simulink model "ComplexPhaseDetectorDual"  (R2016a)
settings: Solver=VariableStepAuto  StartTime=0.0  StopTime=.05  RelTol=1e-6
PreLoadFcn:
  | Bits = 4
  | Ts=2*3/280e6
  | dBRange=11
  | maxNumErrs=500
  | maxNumBits=1e6
  | AM_Gain=AM_GainDiff;
  | AGC_Gain=AGC_GainCalc;
  | load('IIR_Coeffs.mat');
InitFcn:
  | Br= 1/(10*Ts)
  | FreqOffset=00
  | Mode=2
  | BitsPer=[2,2,1,1]
  | EbNo=50
  | N=6
undefined symbols (not defined in the file or in its folder): designMultirateFIR, DiscIntNeverNeededParam
libraries: xbsIndex_r4 x1085, commfilt2 x12, commsink2 x6, dspsigops x5, dspmlti4 x2, commrfcorlib x2, commchan3 x2, dspfdesign x2, dspstat3 x2, commdigbbndpm3 x1, commrandsrc3 x1
(part 2 of 13)

== system ComplexPhaseDetectorDual/AD9957 ==
  In1 : Inport
  Add3 : Sum
  Complex to Real-Imag3 : ComplexToRealImag
  FIR Interpolation : dspmlti4/FIR Interpolation  FilterSource=Auto  h=designMultirateFIR(3,1)  L=8  FilterObject=FINTERP  framing=Allow multirate processing  outputBufInitCond=0  roundingMode=Floor  overflowMode=off  firstCoeffDataTypeStr=Inherit: Same word length as input  firstCoeffMin=[]  firstCoeffMax=[]  firstCoeffLastDataTypeStr=Inherit: Same word length as input  outputDataTypeStr=Inherit: Same as accumulator  outputMin=[]  outputMax=[]  outputLastDataTypeStr=Inherit: Same as accumulator
  NCO : dspsigops/NCO  AccIncSrc=Specify via dialog  AccInc=16384*3/8  PhaseOffsetSrc=Specify via dialog  PhaseOffset=0  AccumWL=16  HasDither=off  DitherWL=4  PNgeneratorLength=19  HasPhaseQuantizer=off  TableDepth=12  HasOutputPhaseError=off  Formula=Sine and cosine  DataType=double  OutputWL=16  OutputFL=14  CompMethod=Table lookup (no interpolation)  SampleTime=Ts/8  SamplesPerFrame=1  OutputFrames=off
  PhaseDetect1 : Product
  PhaseDetect2 : Product
  Out1 : Outport
  wires:
  In1/1 -> FIR Interpolation/1
  NCO/1 -> PhaseDetect2/2
  Complex to Real-Imag3/1 -> PhaseDetect1/1
  PhaseDetect2/1 -> Add3/1
  PhaseDetect1/1 -> Add3/2
  Complex to Real-Imag3/2 -> PhaseDetect2/1
  FIR Interpolation/1 -> Complex to Real-Imag3/1
  NCO/2 -> PhaseDetect1/2
  Add3/1 -> Out1/1

== system ComplexPhaseDetectorDual/AD9957-2 ==
  In1 : Inport
  Add3 : Sum
  Complex to Real-Imag3 : ComplexToRealImag
  FIR Interpolation : dspmlti4/FIR Interpolation  FilterSource=Auto  h=designMultirateFIR(3,1)  L=8  FilterObject=FINTERP  framing=Allow multirate processing  outputBufInitCond=0  roundingMode=Floor  overflowMode=off  firstCoeffDataTypeStr=Inherit: Same word length as input  firstCoeffMin=[]  firstCoeffMax=[]  firstCoeffLastDataTypeStr=Inherit: Same word length as input  outputDataTypeStr=Inherit: Same as accumulator  outputMin=[]  outputMax=[]  outputLastDataTypeStr=Inherit: Same as accumulator
  NCO : dspsigops/NCO  AccIncSrc=Specify via dialog  AccInc=16384*3/8  PhaseOffsetSrc=Specify via dialog  PhaseOffset=0  AccumWL=16  HasDither=off  DitherWL=4  PNgeneratorLength=19  HasPhaseQuantizer=off  TableDepth=12  HasOutputPhaseError=off  Formula=Sine and cosine  DataType=double  OutputWL=16  OutputFL=14  CompMethod=Table lookup (no interpolation)  SampleTime=Ts/8  SamplesPerFrame=1  OutputFrames=off
  PhaseDetect1 : Product
  PhaseDetect2 : Product
  Out1 : Outport
  wires:
  Add3/1 -> Out1/1
  NCO/2 -> PhaseDetect1/2
  FIR Interpolation/1 -> Complex to Real-Imag3/1
  Complex to Real-Imag3/2 -> PhaseDetect2/1
  PhaseDetect1/1 -> Add3/2
  PhaseDetect2/1 -> Add3/1
  Complex to Real-Imag3/1 -> PhaseDetect1/1
  NCO/1 -> PhaseDetect2/2
  In1/1 -> FIR Interpolation/1

== system ComplexPhaseDetectorDual/AGCtoAWGN1 ==
  AGC : Inport
  Bias2 : Bias  Bias=100
  Gain10 : Gain  Gain=3.55
  Gain9 : Gain  Gain=-1/10
  Math Function : Math  Operator=10^u  SaturateOnIntegerOverflow=on
  Variance : Outport
  wires:
  Math Function/1 -> Gain10/1
  Gain10/1 -> Variance/1
  Gain9/1 -> Math Function/1
  Bias2/1 -> Gain9/1
  AGC/1 -> Bias2/1

== system ComplexPhaseDetectorDual/AGCtoAWGN2 ==
  AGC : Inport
  Bias2 : Bias  Bias=100
  Gain10 : Gain  Gain=3.55
  Gain9 : Gain  Gain=-1/10
  Math Function : Math  Operator=10^u  SaturateOnIntegerOverflow=on
  Variance : Outport
  wires:
  AGC/1 -> Bias2/1
  Bias2/1 -> Gain9/1
  Gain9/1 -> Math Function/1
  Gain10/1 -> Variance/1
  Math Function/1 -> Gain10/1

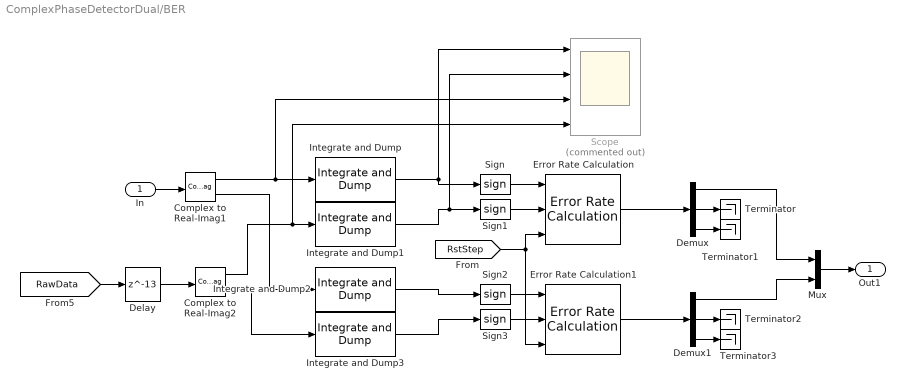
== system ComplexPhaseDetectorDual/BER ==
  In : Inport
  Complex to Real-Imag1 : ComplexToRealImag
  Complex to Real-Imag2 : ComplexToRealImag
  Delay : Delay  DelayLength=13
  Demux : Demux  Outputs=3
  Demux1 : Demux  Outputs=3
  Error Rate Calculation : commsink2/Error Rate Calculation  N=0  st_delay=100  cp_mode=Entire frame  subframe=[]  PMode=Port  WsName=BER  RsMode2=on  stop=off  numErr=maxNumErrs  maxBits=maxNumBits
  Error Rate Calculation1 : commsink2/Error Rate Calculation  N=0  st_delay=100  cp_mode=Entire frame  subframe=[]  PMode=Port  WsName=BER  RsMode2=on  stop=off  numErr=maxNumErrs  maxBits=maxNumBits
  Integrate and Dump{,1..3} (4 alike) : commfilt2/Integrate and Dump  obssamples=1/(Br*Ts)  offsetsamples=3  nodump=off  roundingMode=Floor  overflowMode=off  outputDataTypeStr=Inherit: Same as accumulator  outputLastDataTypeStr=Inherit: Same as accumulator
  Mux : Mux  Inputs=2
  Scope : Scope  Commented=on  NumInputPorts=4
  Sign{,1..3} (4 alike) : Signum
  Terminator{,1..3} (4 alike) : Terminator
  Out1 : Outport
  wires:
  Integrate and Dump1/1 -> Scope/2, Sign1/1
  Error Rate Calculation/1 -> Demux/1
  Integrate and Dump/1 -> Scope/1, Sign/1
  Sign/1 -> Error Rate Calculation/1
  Sign1/1 -> Error Rate Calculation/2
  In/1 -> Complex to Real-Imag1/1
  Complex to Real-Imag2/1 -> Scope/4, Integrate and Dump1/1
  Delay/1 -> Complex to Real-Imag2/1
  [RawData] -> Delay/1
  Complex to Real-Imag1/1 -> Scope/3, Integrate and Dump/1
  Integrate and Dump3/1 -> Sign3/1
  Error Rate Calculation1/1 -> Demux1/1
  Integrate and Dump2/1 -> Sign2/1
  Sign2/1 -> Error Rate Calculation1/1
  Sign3/1 -> Error Rate Calculation1/2
  Complex to Real-Imag2/2 -> Integrate and Dump3/1
  [RstStep] -> Error Rate Calculation1/3, Error Rate Calculation/3
  Complex to Real-Imag1/2 -> Integrate and Dump2/1
  Demux/1 -> Mux/1
  Demux1/1 -> Mux/2
  Demux/2 -> Terminator/1
  Demux/3 -> Terminator1/1
  Demux1/2 -> Terminator2/1
  Demux1/3 -> Terminator3/1
  Mux/1 -> Out1/1

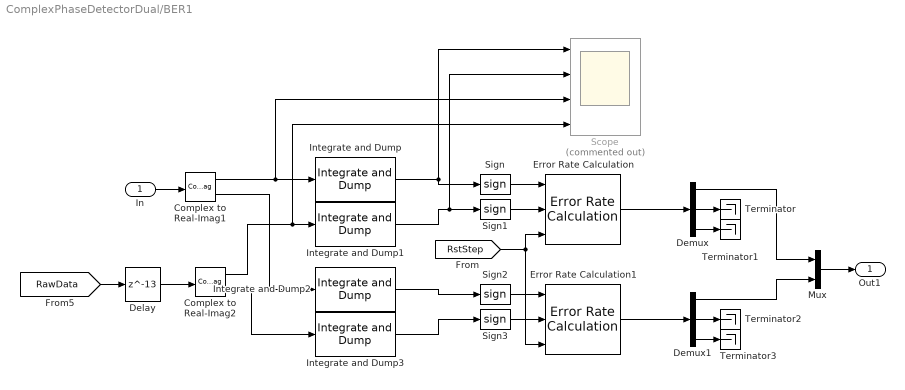
== system ComplexPhaseDetectorDual/BER1 ==
  In : Inport
  Complex to Real-Imag1 : ComplexToRealImag
  Complex to Real-Imag2 : ComplexToRealImag
  Delay : Delay  DelayLength=13
  Demux : Demux  Outputs=3
  Demux1 : Demux  Outputs=3
  Error Rate Calculation : commsink2/Error Rate Calculation  N=0  st_delay=100  cp_mode=Entire frame  subframe=[]  PMode=Port  WsName=BER  RsMode2=on  stop=off  numErr=maxNumErrs  maxBits=maxNumBits
  Error Rate Calculation1 : commsink2/Error Rate Calculation  N=0  st_delay=100  cp_mode=Entire frame  subframe=[]  PMode=Port  WsName=BER  RsMode2=on  stop=off  numErr=maxNumErrs  maxBits=maxNumBits
  Integrate and Dump{,1..3} (4 alike) : commfilt2/Integrate and Dump  obssamples=1/(Br*Ts)  offsetsamples=3  nodump=off  roundingMode=Floor  overflowMode=off  outputDataTypeStr=Inherit: Same as accumulator  outputLastDataTypeStr=Inherit: Same as accumulator
  Mux : Mux  Inputs=2
  Scope : Scope  Commented=on  NumInputPorts=4
  Sign{,1..3} (4 alike) : Signum
  Terminator{,1..3} (4 alike) : Terminator
  Out1 : Outport
  wires:
  Mux/1 -> Out1/1
  Demux1/3 -> Terminator3/1
  Demux1/2 -> Terminator2/1
  Demux/3 -> Terminator1/1
  Demux/2 -> Terminator/1
  Demux1/1 -> Mux/2
  Demux/1 -> Mux/1
  Complex to Real-Imag1/2 -> Integrate and Dump2/1
  [RstStep] -> Error Rate Calculation/3, Error Rate Calculation1/3
  Complex to Real-Imag2/2 -> Integrate and Dump3/1
  Sign3/1 -> Error Rate Calculation1/2
  Sign2/1 -> Error Rate Calculation1/1
  Integrate and Dump2/1 -> Sign2/1
  Error Rate Calculation1/1 -> Demux1/1
  Integrate and Dump3/1 -> Sign3/1
  Complex to Real-Imag1/1 -> Integrate and Dump/1, Scope/3
  [RawData] -> Delay/1
  Delay/1 -> Complex to Real-Imag2/1
  Complex to Real-Imag2/1 -> Integrate and Dump1/1, Scope/4
  In/1 -> Complex to Real-Imag1/1
  Sign1/1 -> Error Rate Calculation/2
  Sign/1 -> Error Rate Calculation/1
  Integrate and Dump/1 -> Sign/1, Scope/1
  Error Rate Calculation/1 -> Demux/1
  Integrate and Dump1/1 -> Sign1/1, Scope/2

== system ComplexPhaseDetectorDual/Conjugate ==
  In1 : Inport
  Complex to Real-Imag : ComplexToRealImag
  Real-Imag to Complex : RealImagToComplex
  Unary Minus : UnaryMinus
  Out1 : Outport
  wires:
  In1/1 -> Complex to Real-Imag/1
  Complex to Real-Imag/1 -> Real-Imag to Complex/1
  Complex to Real-Imag/2 -> Unary Minus/1
  Unary Minus/1 -> Real-Imag to Complex/2
  Real-Imag to Complex/1 -> Out1/1

== system ComplexPhaseDetectorDual/Knob ==

== system ComplexPhaseDetectorDual/LockImag ==
  In : Inport
  Sub : Inport  Port=2
  Rst_n : Inport  Port=3
  Constant : xbsIndex_r4/Constant  const=0  gui_display_data_type=Fixed-point  arith_type=Unsigned  n_bits=13  bin_pt=0  preci_type=Single  exp_width=8  frac_width=24  explicit_period=off  period=1  equ=P=C  opselect=C  inp2=PCIN>>17  opr=+  inp1=P  carry=CIN  dbl_ovrd=off  block_type=constant
  LockReal : xbsIndex_r4/AddSub  mode=Addition or Subtraction  use_carryin=off  use_carryout=off  en=off  latency=1  precision=User Defined  arith_type=Unsigned  n_bits=13  bin_pt=0  quantization=Truncate  overflow=Saturate  use_behavioral_HDL=off  hw_selection=Fabric  pipelined=off  dbl_ovrd=off  block_type=addsub
  Mux : xbsIndex_r4/Mux  inputs=2  en=off  latency=0  precision=Full  arith_type=Unsigned  n_bits=16  bin_pt=14  quantization=Truncate  overflow=Wrap  dbl_ovrd=off  block_type=mux
  Out : Outport
  wires:
  Rst_n/1 -> Mux/1
  Constant/1 -> Mux/2
  Mux/1 -> LockReal/1
  LockReal/1 -> Out/1, Mux/3
  Sub/1 -> LockReal/3
  In/1 -> LockReal/2

== system ComplexPhaseDetectorDual/LockReal ==
  In : Inport
  Sub : Inport  Port=2
  Rst_n : Inport  Port=3
  Constant : xbsIndex_r4/Constant  const=0  gui_display_data_type=Fixed-point  arith_type=Unsigned  n_bits=13  bin_pt=0  preci_type=Single  exp_width=8  frac_width=24  explicit_period=off  period=1  equ=P=C  opselect=C  inp2=PCIN>>17  opr=+  inp1=P  carry=CIN  dbl_ovrd=off  block_type=constant
  LockReal : xbsIndex_r4/AddSub  mode=Addition or Subtraction  use_carryin=off  use_carryout=off  en=off  latency=1  precision=User Defined  arith_type=Unsigned  n_bits=13  bin_pt=0  quantization=Truncate  overflow=Saturate  use_behavioral_HDL=off  hw_selection=Fabric  pipelined=off  dbl_ovrd=off  block_type=addsub
  Mux : xbsIndex_r4/Mux  inputs=2  en=off  latency=0  precision=Full  arith_type=Unsigned  n_bits=16  bin_pt=14  quantization=Truncate  overflow=Wrap  dbl_ovrd=off  block_type=mux
  Out : Outport
  wires:
  In/1 -> LockReal/2
  Sub/1 -> LockReal/3
  LockReal/1 -> Mux/3, Out/1
  Mux/1 -> LockReal/1
  Constant/1 -> Mux/2
  Rst_n/1 -> Mux/1

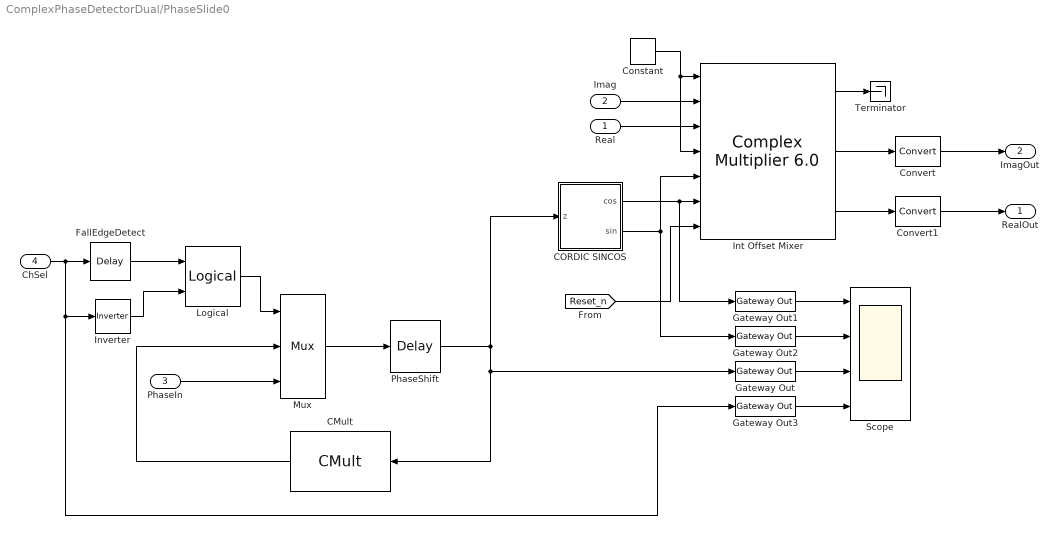
== system ComplexPhaseDetectorDual/PhaseSlide0 ==
  Real : Inport
  Imag : Inport  Port=2
  PhaseIn : Inport  Port=3
  ChSel : Inport  Port=4
  CMult : xbsIndex_r4/CMult  const=.999  gui_display_data_type=Fixed-point  const_n_bits=18  const_bin_pt=17  float_type=Single  exp_bits=8  fraction_bits=24  en=off  latency=1  precision=User Defined  arith_type="Signed  (2's comp)"  n_bits=21  bin_pt=17  quantization=Truncate  overflow=Wrap  use_behavioral_HDL=off  mem_type=Distributed RAM  pipeline=off  dbl_ovrd=off  block_type=cmult
  CORDIC SINCOS : Subsystem  mask(Xilinx CORDIC SINCOS){stages=17, pe_nbits=21, pe_binpt=17, pipeline_x=ones(1,17), prev_stages=17, pipeline=[1  1  1  1  1  1  1  1  1  1  1  1  1  1  1  1  1]}
      mask prompts: stages "Number of Processing Elements (integer value starting from 1)"; pe_nbits "Input Data Width"; pe_binpt "Input Binary Point Position"; pipeline_x "Latency for each Processing Element [1 0 0 1]"; prev_stages "Previous Number of Stages"; pipeline "Previous Pipeline Values"
      mask help: A parallel implementation, circular rotation mode CORDIC processor for calculating Sine and Cosine of input angle z. The number of iteration stages (and resultant output accuracy) and the processor arithmetic precision are controlled by the mask customization.
      mask init:
      | [bg,fg] = xlcmap('XBlock',0);
      | iPos = get_param(gcb,'Position');
      | iWidth=iPos(3)-iPos(1); iHeight=iPos(4)-iPos(2);
      | iCx=iWidth/2;
      | iCy=iHeight/2;
      | [logoX, logoY] = xlogo(iPos);
      | sav_gcb=gcb;
      | stages = round(sum(abs(stages)));
      | if (stages == 0)
      | 	stages = prev_stages;
      | end
      | x = zeros(1,stages);
      | pipe_size = max(size(pipeline_x));
      | if pipe_size >= stages
      | 	x(1,1:stages) = pipeline_x(1,1:stages);
      | else
      | 	x(1,1:pipe_size) = pipeline_x(1,1:pipe_size);
      | end
      | 
      | if (stages ~=prev_stages)
      | 	pipeline=x;
      | 	cordic_pe = find_system(gcb, 'lookUnderMasks', 'all', 'FollowLinks','on','masktype', 'CORDIC parallel PE');
      |     
      |   a=find_system(cordic_pe{1}, 'lookUnderMasks', 'all', 'FollowLinks','on','masktype', 'CORDIC iteration PE');
      |   for i= 2:length(a)
      |     for j=1:3
      | 	  delete_line(cordic_pe{1}, ['CORDIC PE' int2str(i-1) '/' int2str(j)], ['CORDIC PE' int2str(i) '/' int2str(j)]);
      |     end
      |   end
      |     if length(a)>0,
      |       delete_line(cordic_pe{1}, 'x/1', 'CORDIC PE1/1');
      |       delete_line(cordic_pe{1}, 'y/1', 'CORDIC PE1/2');
      |       delete_line(cordic_pe{1}, 'z/1', 'CORDIC PE1/3');
      |       delete_line(cordic_pe{1}, ['CORDIC PE' int2str(length(a)) '/1'],'X/1');
      |       delete_line(cordic_pe{1}, ['CORDIC PE' int2str(length(a)) '/2'],'Y/1');
      |       delete_line(cordic_pe{1}, ['CORDIC PE' int2str(length(a)) '/3'],'Terminator/1');
      |     elseif length(a)==0
      |       temp_port=get_param([cordic_pe{1} '/x'],'porthandles');
      |       temp_line=get_param(temp_port.Outport,'line');
      |       if temp_line>=0  delete_line(temp_line); end
      |       temp_port=get_param([cordic_pe{1} '/y'],'porthandles');
      |       temp_line=get_param(temp_port.Outport,'line');
      |       if temp_line>=0  delete_line(temp_line); end
      |       temp_port=get_param([cordic_pe{1} '/z'],'porthandles');
      |       temp_line=get_param(temp_port.Outport,'line');
      |       if temp_line>=0  delete_line(temp_line); end
      |     end
      | 
      |     for i=2:length(a)
      |       delete_block(a{i});
      |     end
      |     for i=2:stages,
      |         add_block([cordic_pe{1} '/CORDIC PE1'], [cordic_pe{1} '/CORDIC PE' int2str(i)], 'ii', int2str(i-1),'pe_nbits', 'pe_nbits','pe_binpt', 'pe_binpt','pipeline',['pipeline(1,' int2str(i) ')'],'position',[150+(i-1)*125, 70, 205+(i-1)*125, 130]);
      |     end
      | 
      |     for i= 2:stages,
      |       for j=1:3
      | 		add_line(cordic_pe{1}, ['CORDIC PE' int2str(i-1) '/' int2str(j)], ['CORDIC PE' int2str(i) '/' int2str(j)], 'autorouting', 'on');
      |       end
      |     end
      | 
      |     if stages==0
      |       add_line(cordic_pe{1}, 'x/1', 'X/1', 'autorouting', 'on');
      |       add_line(cordic_pe{1}, 'y/1', 'Terminator/1', 'autorouting', 'on');
      |       add_line(cordic_pe{1}, 'z/1', 'Z/1', 'autorouting', 'on');
      |     elseif stages>0
      |       add_line(cordic_pe{1}, 'x/1', 'CORDIC PE1/1', 'autorouting', 'on');
      |       add_line(cordic_pe{1}, 'y/1', 'CORDIC PE1/2', 'autorouting', 'on');
      |       add_line(cordic_pe{1}, 'z/1', 'CORDIC PE1/3', 'autorouting', 'on');
      | 
      |       set_param([cordic_pe{1} '/' 'X'], 'Position', [150+stages*125, 72, 180+stages*125, 86]);
      |       set_param([cordic_pe{1} '/' 'Y'], 'Position', [210+stages*125, 92, 225+stages*125, 108]);
      |       set_param([cordic_pe{1} '/' 'Terminator'], 'Position', [240+stages*125, 113, 270+stages*125, 127]);
      | 
      |       add_line(cordic_pe{1}, ['CORDIC PE' int2str(stages) '/1'], 'X/1', 'autorouting', 'on');
      |       add_line(cordic_pe{1}, ['CORDIC PE' int2str(stages) '/2'], 'Y/1', 'autorouting', 'on');
      |       add_line(cordic_pe{1}, ['CORDIC PE' int2str(stages) '/3'],'Terminator/1', 'autorouting', 'on');
      | 
      |       % force a "compile" of the constituent constant blocks to
      |       % workaround a data propagation problem
      |       find_system(cordic_pe{1}, 'lookUnderMasks', 'all', 'FollowLinks', 'on', 'MaskType','Xilinx Constant Block');
      |   end
      | 	set_param(sav_gcb, 'prev_stages', int2str(stages));
      | 	set_param(sav_gcb, 'pipeline', [ '[' int2str(x) ']']);
      | else
      | 	if (sum(pipeline~=x))
      | 		set_param(gcb, 'pipeline', [ '[' int2str(x) ']']);
      | 	end
      | end
      | str = sprintf('-%d',sum(x) + 3);
      settings: CopyFcn=set_param(gcb, 'MaskSelfModifiable', 'on', 'LinkStatus', 'none');
      mask Help: eval('');xlDoc('-book','sysgen','-topic','CORDIC_SINCOS');
      mask Display:
      | patch([0 iWidth iWidth 0],[0 0 iHeight iHeight] , bg);
      | patch(logoX,logoY , fg);
      | text(iCx-6,iCy,'z');
      | text(iCx,iCy+4,str);
      | port_label('input',1,'z');
      | port_label('output',1,'cos');
      | port_label('output',2,'sin');
      | plot([0 0 iWidth iWidth 0], [0 iHeight iHeight 0 0]);
  Constant : xbsIndex_r4/Constant  const=1  gui_display_data_type=Boolean  arith_type=Boolean  n_bits=16  bin_pt=14  preci_type=Single  exp_width=8  frac_width=24  explicit_period=on  period=Ts  equ=P=C  opselect=C  inp2=PCIN>>17  opr=+  inp1=P  carry=CIN  dbl_ovrd=off  block_type=constant
  Convert : xbsIndex_r4/Convert  gui_display_data_type=Fixed-point  arith_type="Signed  (2's comp)"  n_bits=18  bin_pt=17  float_type=Single  exp_bits=8  fraction_bits=24  quantization=Truncate  overflow=Saturate  en=off  latency=1  pipeline=off  dbl_ovrd=off  block_type=convert
  Convert1 : xbsIndex_r4/Convert  gui_display_data_type=Fixed-point  arith_type="Signed  (2's comp)"  n_bits=18  bin_pt=17  float_type=Single  exp_bits=8  fraction_bits=24  quantization=Truncate  overflow=Saturate  en=off  latency=1  pipeline=off  dbl_ovrd=off  block_type=convert
  FallEdgeDetect : xbsIndex_r4/Delay  rst=off  infoeditControl=Selection of Reset will increase slice count due to use of real FFs and instead of SRLs  en=off  latency=4  reg_retiming=off  dbl_ovrd=off  block_type=delay
  Gateway Out{,1..3} (4 alike) : xbsIndex_r4/Gateway Out  inherit_from_input=off  hdl_port=off  rows=1  columns=1  UseAsDAC=off  DACChannel='1'  interface=None  automatic_assignment=on  address_offset=hex2dec('00')  intf_name=''  intf_description=''  timing_constraint=None  locs_specified=off  LOCs={}  io_standard={}  block_type=gatewayout
  Int Offset Mixer : xbsIndex_r4/Complex Multiplier 6.0   hasatlast=off  hasatuser=off  atuserwidth=1  hasbtlast=off  hasbtuser=off  btuserwidth=1  multtype=Use_Mults  optimizegoal=Resources  flowcontrol=NonBlocking  outputwidth=20  roundmode=Truncate  hasctrltlast=off  hasctrltuser=off  ctrltuserwidth=1  outtlastbehv=Null  latencyconfig=Manual  minimumlatency=3  aclken=off  aresetn=on  trim_axipin_name=on  simulation_type=hybrid_sim  simulation_model=sysgen:cmpy_v6_0  data_path_portlist={ 's_axis_a_tdata_real', 's_axis_a_tdata_imag', 's_axis_b_tdata_real', 's_axis_b_tdata_imag', 's_axis_ctrl_tdata_rounding_bit', 'm_axis_dout_tdata_real', 'm_axis_dout_tdata_imag' }  aportwidth=63  bportwidth=63  ip_name=Complex Multiplier  ip_version=6.0  dsptool_ready=true  ipcore_usecache=true  ipcore_useipmodelcache=true  ipcore_verbose=false  ipcore_latency_parameter='minimumlatency'  wrapper_available=true  port_translation_map={ 'aclken' => 'en', 'aresetn' => 'rst'}  block_type=cmpy_v6_0
  Inverter : xbsIndex_r4/Inverter  en=off  latency=0  dbl_ovrd=off  block_type=inv
  Logical : xbsIndex_r4/Logical  logical_function=AND  inputs=2  en=off  latency=0  precision=Full  arith_type=Unsigned  n_bits=16  bin_pt=0  align_bp=on  dbl_ovrd=off  block_type=logical
  Mux : xbsIndex_r4/Mux  inputs=2  en=off  latency=0  precision=Full  arith_type=Unsigned  n_bits=16  bin_pt=14  quantization=Truncate  overflow=Wrap  dbl_ovrd=off  block_type=mux
  PhaseShift : xbsIndex_r4/Delay  rst=off  infoeditControl=Selection of Reset will increase slice count due to use of real FFs and instead of SRLs  en=off  latency=1  reg_retiming=off  dbl_ovrd=off  block_type=delay
  Scope : Scope  NumInputPorts=4
  Terminator : Terminator
  RealOut : Outport
  ImagOut : Outport  Port=2
  wires:
  Imag/1 -> Int Offset Mixer/2
  Constant/1 -> Int Offset Mixer/4, Int Offset Mixer/1
  CORDIC SINCOS/2(sin) -> Int Offset Mixer/5, Gateway Out2/1
  Int Offset Mixer/1 -> Terminator/1
  Convert1/1 -> RealOut/1
  Real/1 -> Int Offset Mixer/3
  Convert/1 -> ImagOut/1
  CORDIC SINCOS/1(cos) -> Int Offset Mixer/6, Gateway Out1/1
  Mux/1 -> PhaseShift/1
  CMult/1 -> Mux/2
  PhaseIn/1 -> Mux/3
  ChSel/1 -> Gateway Out3/1, Inverter/1, FallEdgeDetect/1
  Logical/1 -> Mux/1
  FallEdgeDetect/1 -> Logical/1
  Inverter/1 -> Logical/2
  Gateway Out1/1 -> Scope/1
  Gateway Out2/1 -> Scope/2
  Gateway Out/1 -> Scope/3
  PhaseShift/1 -> CMult/1, Gateway Out/1, CORDIC SINCOS/1(z)
  Int Offset Mixer/3 -> Convert1/1
  Int Offset Mixer/2 -> Convert/1
  [Reset_n] -> Int Offset Mixer/7
  Gateway Out3/1 -> Scope/4

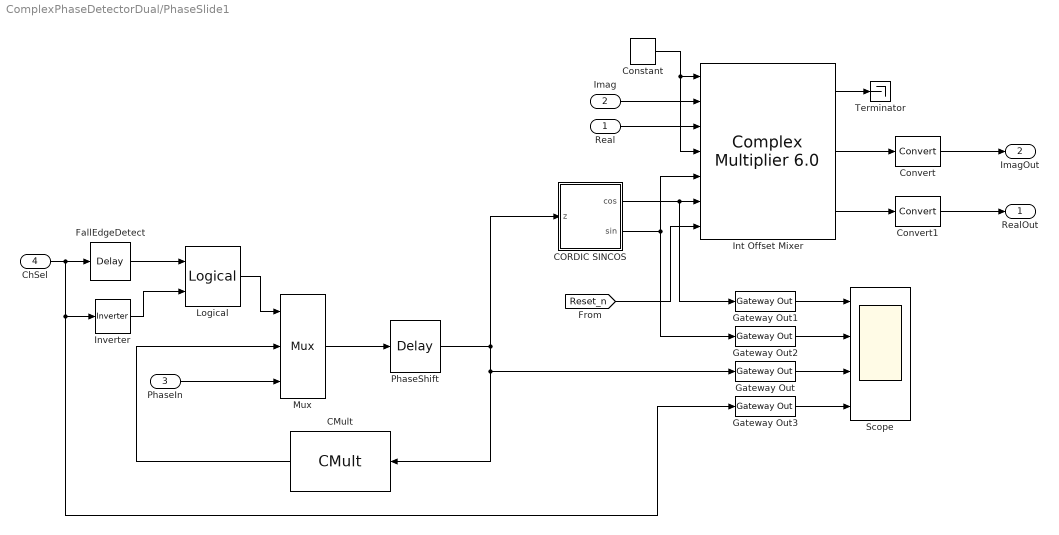
== system ComplexPhaseDetectorDual/PhaseSlide1 ==
  Real : Inport
  Imag : Inport  Port=2
  PhaseIn : Inport  Port=3
  ChSel : Inport  Port=4
  CMult : xbsIndex_r4/CMult  const=.999  gui_display_data_type=Fixed-point  const_n_bits=18  const_bin_pt=17  float_type=Single  exp_bits=8  fraction_bits=24  en=off  latency=1  precision=User Defined  arith_type="Signed  (2's comp)"  n_bits=21  bin_pt=17  quantization=Truncate  overflow=Wrap  use_behavioral_HDL=off  mem_type=Distributed RAM  pipeline=off  dbl_ovrd=off  block_type=cmult
  CORDIC SINCOS : Subsystem  mask(Xilinx CORDIC SINCOS){stages=17, pe_nbits=21, pe_binpt=17, pipeline_x=ones(1,17), prev_stages=17, pipeline=[1  1  1  1  1  1  1  1  1  1  1  1  1  1  1  1  1]}
      mask prompts: stages "Number of Processing Elements (integer value starting from 1)"; pe_nbits "Input Data Width"; pe_binpt "Input Binary Point Position"; pipeline_x "Latency for each Processing Element [1 0 0 1]"; prev_stages "Previous Number of Stages"; pipeline "Previous Pipeline Values"
      mask help: A parallel implementation, circular rotation mode CORDIC processor for calculating Sine and Cosine of input angle z. The number of iteration stages (and resultant output accuracy) and the processor arithmetic precision are controlled by the mask customization.
      mask init: same as ComplexPhaseDetectorDual/PhaseSlide0/CORDIC SINCOS
      settings: CopyFcn=set_param(gcb, 'MaskSelfModifiable', 'on', 'LinkStatus', 'none');
      mask Help: eval('');xlDoc('-book','sysgen','-topic','CORDIC_SINCOS');
      mask Display:
      | patch([0 iWidth iWidth 0],[0 0 iHeight iHeight] , bg);
      | patch(logoX,logoY , fg);
      | text(iCx-6,iCy,'z');
      | text(iCx,iCy+4,str);
      | port_label('input',1,'z');
      | port_label('output',1,'cos');
      | port_label('output',2,'sin');
      | plot([0 0 iWidth iWidth 0], [0 iHeight iHeight 0 0]);
  Constant : xbsIndex_r4/Constant  const=1  gui_display_data_type=Boolean  arith_type=Boolean  n_bits=16  bin_pt=14  preci_type=Single  exp_width=8  frac_width=24  explicit_period=on  period=Ts  equ=P=C  opselect=C  inp2=PCIN>>17  opr=+  inp1=P  carry=CIN  dbl_ovrd=off  block_type=constant
  Convert : xbsIndex_r4/Convert  gui_display_data_type=Fixed-point  arith_type="Signed  (2's comp)"  n_bits=18  bin_pt=17  float_type=Single  exp_bits=8  fraction_bits=24  quantization=Truncate  overflow=Saturate  en=off  latency=1  pipeline=off  dbl_ovrd=off  block_type=convert
  Convert1 : xbsIndex_r4/Convert  gui_display_data_type=Fixed-point  arith_type="Signed  (2's comp)"  n_bits=18  bin_pt=17  float_type=Single  exp_bits=8  fraction_bits=24  quantization=Truncate  overflow=Saturate  en=off  latency=1  pipeline=off  dbl_ovrd=off  block_type=convert
  FallEdgeDetect : xbsIndex_r4/Delay  rst=off  infoeditControl=Selection of Reset will increase slice count due to use of real FFs and instead of SRLs  en=off  latency=4  reg_retiming=off  dbl_ovrd=off  block_type=delay
  Gateway Out{,1..3} (4 alike) : xbsIndex_r4/Gateway Out  inherit_from_input=off  hdl_port=off  rows=1  columns=1  UseAsDAC=off  DACChannel='1'  interface=None  automatic_assignment=on  address_offset=hex2dec('00')  intf_name=''  intf_description=''  timing_constraint=None  locs_specified=off  LOCs={}  io_standard={}  block_type=gatewayout
  Int Offset Mixer : xbsIndex_r4/Complex Multiplier 6.0   hasatlast=off  hasatuser=off  atuserwidth=1  hasbtlast=off  hasbtuser=off  btuserwidth=1  multtype=Use_Mults  optimizegoal=Resources  flowcontrol=NonBlocking  outputwidth=20  roundmode=Truncate  hasctrltlast=off  hasctrltuser=off  ctrltuserwidth=1  outtlastbehv=Null  latencyconfig=Manual  minimumlatency=3  aclken=off  aresetn=on  trim_axipin_name=on  simulation_type=hybrid_sim  simulation_model=sysgen:cmpy_v6_0  data_path_portlist={ 's_axis_a_tdata_real', 's_axis_a_tdata_imag', 's_axis_b_tdata_real', 's_axis_b_tdata_imag', 's_axis_ctrl_tdata_rounding_bit', 'm_axis_dout_tdata_real', 'm_axis_dout_tdata_imag' }  aportwidth=63  bportwidth=63  ip_name=Complex Multiplier  ip_version=6.0  dsptool_ready=true  ipcore_usecache=true  ipcore_useipmodelcache=true  ipcore_verbose=false  ipcore_latency_parameter='minimumlatency'  wrapper_available=true  port_translation_map={ 'aclken' => 'en', 'aresetn' => 'rst'}  block_type=cmpy_v6_0
  Inverter : xbsIndex_r4/Inverter  en=off  latency=0  dbl_ovrd=off  block_type=inv
  Logical : xbsIndex_r4/Logical  logical_function=AND  inputs=2  en=off  latency=0  precision=Full  arith_type=Unsigned  n_bits=16  bin_pt=0  align_bp=on  dbl_ovrd=off  block_type=logical
  Mux : xbsIndex_r4/Mux  inputs=2  en=off  latency=0  precision=Full  arith_type=Unsigned  n_bits=16  bin_pt=14  quantization=Truncate  overflow=Wrap  dbl_ovrd=off  block_type=mux
  PhaseShift : xbsIndex_r4/Delay  rst=off  infoeditControl=Selection of Reset will increase slice count due to use of real FFs and instead of SRLs  en=off  latency=1  reg_retiming=off  dbl_ovrd=off  block_type=delay
  Scope : Scope  NumInputPorts=4
  Terminator : Terminator
  RealOut : Outport
  ImagOut : Outport  Port=2
  wires:
  Gateway Out3/1 -> Scope/4
  [Reset_n] -> Int Offset Mixer/7
  Int Offset Mixer/2 -> Convert/1
  Int Offset Mixer/3 -> Convert1/1
  PhaseShift/1 -> CORDIC SINCOS/1(z), Gateway Out/1, CMult/1
  Gateway Out/1 -> Scope/3
  Gateway Out2/1 -> Scope/2
  Gateway Out1/1 -> Scope/1
  Inverter/1 -> Logical/2
  FallEdgeDetect/1 -> Logical/1
  Logical/1 -> Mux/1
  ChSel/1 -> FallEdgeDetect/1, Inverter/1, Gateway Out3/1
  PhaseIn/1 -> Mux/3
  CMult/1 -> Mux/2
  Mux/1 -> PhaseShift/1
  CORDIC SINCOS/1(cos) -> Gateway Out1/1, Int Offset Mixer/6
  Convert/1 -> ImagOut/1
  Real/1 -> Int Offset Mixer/3
  Convert1/1 -> RealOut/1
  Int Offset Mixer/1 -> Terminator/1
  CORDIC SINCOS/2(sin) -> Gateway Out2/1, Int Offset Mixer/5
  Constant/1 -> Int Offset Mixer/1, Int Offset Mixer/4
  Imag/1 -> Int Offset Mixer/2

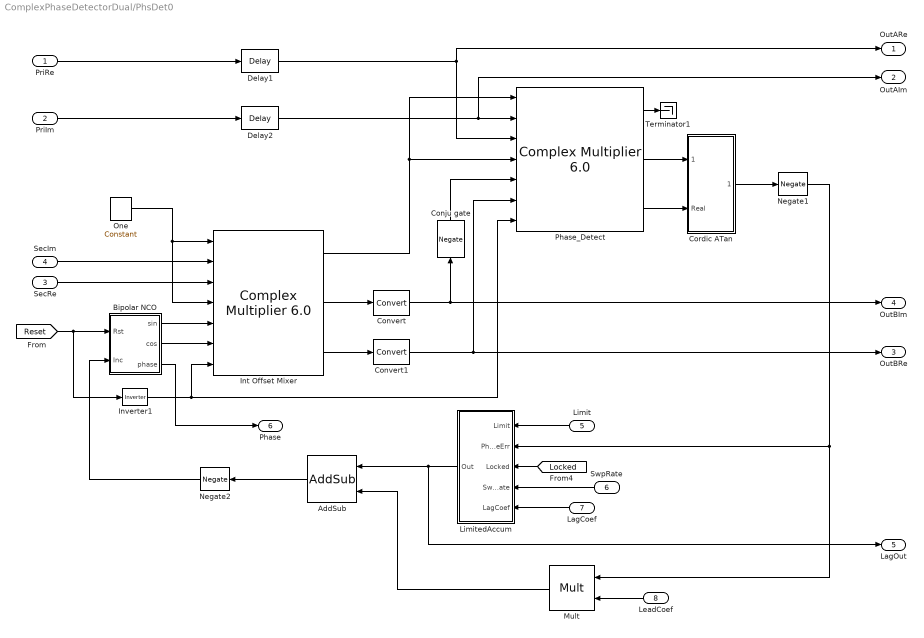
== system ComplexPhaseDetectorDual/PhsDet0 ==
  PriRe : Inport
  PriIm : Inport  Port=2
  SecRe : Inport  Port=3
  SecIm : Inport  Port=4
  Limit : Inport  Port=5
  SwpRate : Inport  Port=6
  LagCoef : Inport  Port=7
  LeadCoef : Inport  Port=8
  AddSub : xbsIndex_r4/AddSub  mode=Addition  use_carryin=off  use_carryout=off  en=off  latency=1  precision=User Defined  arith_type="Signed  (2's comp)"  n_bits=18+Bits  bin_pt=0  quantization=Truncate  overflow=Wrap  use_behavioral_HDL=off  hw_selection=Fabric  pipelined=off  dbl_ovrd=off  block_type=addsub
  Bipolar NCO : Subsystem
  Conju gate : xbsIndex_r4/Negate  precision=User Defined  arith_type="Signed  (2's comp)"  n_bits=18  bin_pt=17  quantization=Truncate  overflow=Saturate  en=off  latency=0  dbl_ovrd=off  block_type=negate
  Convert : xbsIndex_r4/Convert  gui_display_data_type=Fixed-point  arith_type="Signed  (2's comp)"  n_bits=18  bin_pt=17  float_type=Single  exp_bits=8  fraction_bits=24  quantization=Truncate  overflow=Saturate  en=off  latency=1  pipeline=off  dbl_ovrd=off  block_type=convert
  Convert1 : xbsIndex_r4/Convert  gui_display_data_type=Fixed-point  arith_type="Signed  (2's comp)"  n_bits=18  bin_pt=17  float_type=Single  exp_bits=8  fraction_bits=24  quantization=Truncate  overflow=Saturate  en=off  latency=1  pipeline=off  dbl_ovrd=off  block_type=convert
  Cordic ATan : Subsystem
  Delay1 : xbsIndex_r4/Delay  rst=off  infoeditControl=Selection of Reset will increase slice count due to use of real FFs and instead of SRLs  en=off  latency=4  reg_retiming=off  dbl_ovrd=off  block_type=delay
  Delay2 : xbsIndex_r4/Delay  rst=off  infoeditControl=Selection of Reset will increase slice count due to use of real FFs and instead of SRLs  en=off  latency=4  reg_retiming=off  dbl_ovrd=off  block_type=delay
  Int Offset Mixer : xbsIndex_r4/Complex Multiplier 6.0   hasatlast=off  hasatuser=off  atuserwidth=1  hasbtlast=off  hasbtuser=off  btuserwidth=1  multtype=Use_Mults  optimizegoal=Resources  flowcontrol=NonBlocking  outputwidth=20  roundmode=Truncate  hasctrltlast=off  hasctrltuser=off  ctrltuserwidth=1  outtlastbehv=Null  latencyconfig=Manual  minimumlatency=3  aclken=off  aresetn=on  trim_axipin_name=on  simulation_type=hybrid_sim  simulation_model=sysgen:cmpy_v6_0  data_path_portlist={ 's_axis_a_tdata_real', 's_axis_a_tdata_imag', 's_axis_b_tdata_real', 's_axis_b_tdata_imag', 's_axis_ctrl_tdata_rounding_bit', 'm_axis_dout_tdata_real', 'm_axis_dout_tdata_imag' }  aportwidth=63  bportwidth=63  ip_name=Complex Multiplier  ip_version=6.0  dsptool_ready=true  ipcore_usecache=true  ipcore_useipmodelcache=true  ipcore_verbose=false  ipcore_latency_parameter='minimumlatency'  wrapper_available=true  port_translation_map={ 'aclken' => 'en', 'aresetn' => 'rst'}  block_type=cmpy_v6_0
  Inverter1 : xbsIndex_r4/Inverter  en=off  latency=0  dbl_ovrd=off  block_type=inv
  LimitedAccum : Subsystem
  Mult : xbsIndex_r4/Mult  precision=User Defined  arith_type="Signed  (2's comp)"  n_bits=18+Bits  bin_pt=9  quantization="Round  (unbiased: +/- Inf)"  overflow=Wrap  en=off  latency=4  use_behavioral_HDL=off  opt=Speed  use_embedded=on  optimum_pipeline=off  pipeline=on  dbl_ovrd=off  use_rpm=on  placement_style=Triangular  block_type=mult
  Negate1 : xbsIndex_r4/Negate  precision=User Defined  arith_type="Signed  (2's comp)"  n_bits=18  bin_pt=15  quantization=Truncate  overflow=Saturate  en=off  latency=0  dbl_ovrd=off  block_type=negate
  Negate2 : xbsIndex_r4/Negate  precision=User Defined  arith_type="Signed  (2's comp)"  n_bits=22  bin_pt=0  quantization=Truncate  overflow=Saturate  en=off  latency=0  dbl_ovrd=off  block_type=negate
  One : xbsIndex_r4/Constant  const=1  gui_display_data_type=Boolean  arith_type=Boolean  n_bits=18  bin_pt=17  preci_type=Single  exp_width=8  frac_width=24  explicit_period=on  period=Ts  equ=P=C  opselect=C  inp2=PCIN>>17  opr=+  inp1=P  carry=CIN  dbl_ovrd=off  block_type=constant
  Phase_Detect : xbsIndex_r4/Complex Multiplier 6.0   hasatlast=off  hasatuser=off  atuserwidth=1  hasbtlast=off  hasbtuser=off  btuserwidth=1  multtype=Use_Mults  optimizegoal=Resources  flowcontrol=NonBlocking  outputwidth=18  roundmode=Truncate  hasctrltlast=off  hasctrltuser=off  ctrltuserwidth=1  outtlastbehv=Null  latencyconfig=Automatic  minimumlatency=37  aclken=off  aresetn=on  trim_axipin_name=on  simulation_type=hybrid_sim  simulation_model=sysgen:cmpy_v6_0  data_path_portlist={ 's_axis_a_tdata_real', 's_axis_a_tdata_imag', 's_axis_b_tdata_real', 's_axis_b_tdata_imag', 's_axis_ctrl_tdata_rounding_bit', 'm_axis_dout_tdata_real', 'm_axis_dout_tdata_imag' }  aportwidth=63  bportwidth=63  ip_name=Complex Multiplier  ip_version=6.0  dsptool_ready=true  ipcore_usecache=true  ipcore_useipmodelcache=true  ipcore_verbose=false  ipcore_latency_parameter='minimumlatency'  wrapper_available=true  port_translation_map={ 'aclken' => 'en', 'aresetn' => 'rst'}  block_type=cmpy_v6_0
  Terminator1 : Terminator
  OutARe : Outport
  OutAIm : Outport  Port=2
  OutBRe : Outport  Port=3
  OutBIm : Outport  Port=4
  LagOut : Outport  Port=5
  Phase : Outport  Port=6
  wires:
  Negate2/1 -> Bipolar NCO/2(Inc)
  Inverter1/1 -> Int Offset Mixer/7, Phase_Detect/7
  [Reset] -> Bipolar NCO/1(Rst), Inverter1/1
  [Locked] -> LimitedAccum/3(Locked)
  SwpRate/1 -> LimitedAccum/4(SwpRate)
  Negate1/1 -> LimitedAccum/2(PhaseErr), Mult/1
  LimitedAccum/1(Out) -> LagOut/1, AddSub/1
  Cordic ATan/1(Phase) -> Negate1/1
  AddSub/1 -> Negate2/1
  Delay1/1 -> OutARe/1, Phase_Detect/3
  PriIm/1 -> Delay2/1
  PriRe/1 -> Delay1/1
  SecIm/1 -> Int Offset Mixer/2
  Limit/1 -> LimitedAccum/1(Limit)
  SecRe/1 -> Int Offset Mixer/3
  Delay2/1 -> OutAIm/1, Phase_Detect/2
  Phase_Detect/2 -> Cordic ATan/1(Imag)
  Phase_Detect/3 -> Cordic ATan/2(Real)
  Bipolar NCO/1(sin) -> Int Offset Mixer/5
  Int Offset Mixer/3 -> Convert1/1
  Convert/1 -> Conju gate/1, OutBIm/1
  Phase_Detect/1 -> Terminator1/1
  Convert1/1 -> Phase_Detect/6, OutBRe/1
  Mult/1 -> AddSub/2
  One/1 -> Int Offset Mixer/4, Int Offset Mixer/1
  Bipolar NCO/2(cos) -> Int Offset Mixer/6
  LeadCoef/1 -> Mult/2
  LagCoef/1 -> LimitedAccum/5(LagCoef)
  Conju gate/1 -> Phase_Detect/5
  Int Offset Mixer/1 -> Phase_Detect/1, Phase_Detect/4
  Int Offset Mixer/2 -> Convert/1
  Bipolar NCO/3(phase) -> Phase/1

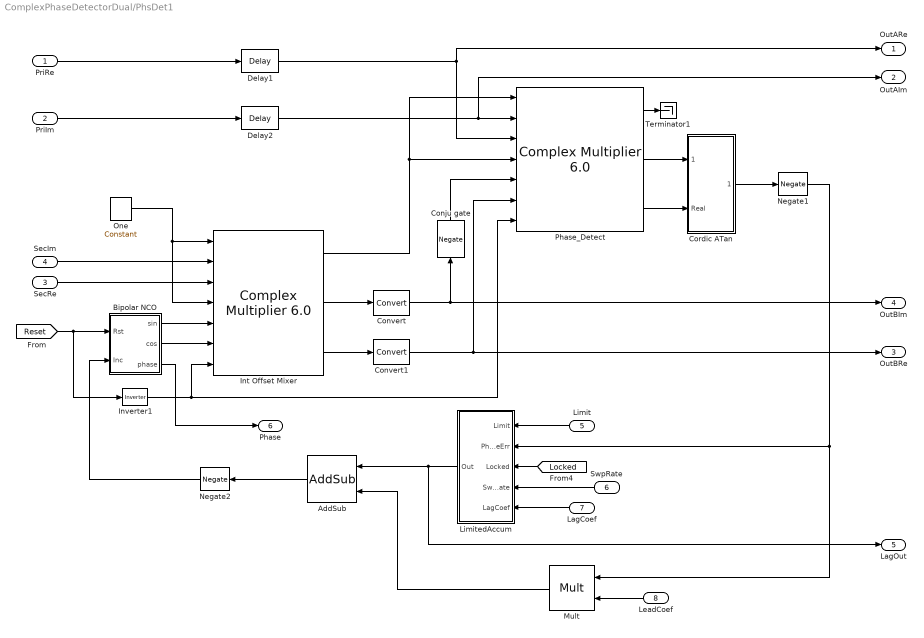
== system ComplexPhaseDetectorDual/PhsDet1 ==
  PriRe : Inport
  PriIm : Inport  Port=2
  SecRe : Inport  Port=3
  SecIm : Inport  Port=4
  Limit : Inport  Port=5
  SwpRate : Inport  Port=6
  LagCoef : Inport  Port=7
  LeadCoef : Inport  Port=8
  AddSub : xbsIndex_r4/AddSub  mode=Addition  use_carryin=off  use_carryout=off  en=off  latency=1  precision=User Defined  arith_type="Signed  (2's comp)"  n_bits=18+Bits  bin_pt=0  quantization=Truncate  overflow=Wrap  use_behavioral_HDL=off  hw_selection=Fabric  pipelined=off  dbl_ovrd=off  block_type=addsub
  Bipolar NCO : Subsystem
  Conju gate : xbsIndex_r4/Negate  precision=User Defined  arith_type="Signed  (2's comp)"  n_bits=18  bin_pt=17  quantization=Truncate  overflow=Saturate  en=off  latency=0  dbl_ovrd=off  block_type=negate
  Convert : xbsIndex_r4/Convert  gui_display_data_type=Fixed-point  arith_type="Signed  (2's comp)"  n_bits=18  bin_pt=17  float_type=Single  exp_bits=8  fraction_bits=24  quantization=Truncate  overflow=Saturate  en=off  latency=1  pipeline=off  dbl_ovrd=off  block_type=convert
  Convert1 : xbsIndex_r4/Convert  gui_display_data_type=Fixed-point  arith_type="Signed  (2's comp)"  n_bits=18  bin_pt=17  float_type=Single  exp_bits=8  fraction_bits=24  quantization=Truncate  overflow=Saturate  en=off  latency=1  pipeline=off  dbl_ovrd=off  block_type=convert
  Cordic ATan : Subsystem
  Delay1 : xbsIndex_r4/Delay  rst=off  infoeditControl=Selection of Reset will increase slice count due to use of real FFs and instead of SRLs  en=off  latency=4  reg_retiming=off  dbl_ovrd=off  block_type=delay
  Delay2 : xbsIndex_r4/Delay  rst=off  infoeditControl=Selection of Reset will increase slice count due to use of real FFs and instead of SRLs  en=off  latency=4  reg_retiming=off  dbl_ovrd=off  block_type=delay
  Int Offset Mixer : xbsIndex_r4/Complex Multiplier 6.0   hasatlast=off  hasatuser=off  atuserwidth=1  hasbtlast=off  hasbtuser=off  btuserwidth=1  multtype=Use_Mults  optimizegoal=Resources  flowcontrol=NonBlocking  outputwidth=20  roundmode=Truncate  hasctrltlast=off  hasctrltuser=off  ctrltuserwidth=1  outtlastbehv=Null  latencyconfig=Manual  minimumlatency=3  aclken=off  aresetn=on  trim_axipin_name=on  simulation_type=hybrid_sim  simulation_model=sysgen:cmpy_v6_0  data_path_portlist={ 's_axis_a_tdata_real', 's_axis_a_tdata_imag', 's_axis_b_tdata_real', 's_axis_b_tdata_imag', 's_axis_ctrl_tdata_rounding_bit', 'm_axis_dout_tdata_real', 'm_axis_dout_tdata_imag' }  aportwidth=63  bportwidth=63  ip_name=Complex Multiplier  ip_version=6.0  dsptool_ready=true  ipcore_usecache=true  ipcore_useipmodelcache=true  ipcore_verbose=false  ipcore_latency_parameter='minimumlatency'  wrapper_available=true  port_translation_map={ 'aclken' => 'en', 'aresetn' => 'rst'}  block_type=cmpy_v6_0
  Inverter1 : xbsIndex_r4/Inverter  en=off  latency=0  dbl_ovrd=off  block_type=inv
  LimitedAccum : Subsystem
  Mult : xbsIndex_r4/Mult  precision=User Defined  arith_type="Signed  (2's comp)"  n_bits=18+Bits  bin_pt=9  quantization="Round  (unbiased: +/- Inf)"  overflow=Wrap  en=off  latency=4  use_behavioral_HDL=off  opt=Speed  use_embedded=on  optimum_pipeline=off  pipeline=on  dbl_ovrd=off  use_rpm=on  placement_style=Triangular  block_type=mult
  Negate1 : xbsIndex_r4/Negate  precision=User Defined  arith_type="Signed  (2's comp)"  n_bits=18  bin_pt=15  quantization=Truncate  overflow=Saturate  en=off  latency=0  dbl_ovrd=off  block_type=negate
  Negate2 : xbsIndex_r4/Negate  precision=User Defined  arith_type="Signed  (2's comp)"  n_bits=22  bin_pt=0  quantization=Truncate  overflow=Saturate  en=off  latency=0  dbl_ovrd=off  block_type=negate
  One : xbsIndex_r4/Constant  const=1  gui_display_data_type=Boolean  arith_type=Boolean  n_bits=18  bin_pt=17  preci_type=Single  exp_width=8  frac_width=24  explicit_period=on  period=Ts  equ=P=C  opselect=C  inp2=PCIN>>17  opr=+  inp1=P  carry=CIN  dbl_ovrd=off  block_type=constant
  Phase_Detect : xbsIndex_r4/Complex Multiplier 6.0   hasatlast=off  hasatuser=off  atuserwidth=1  hasbtlast=off  hasbtuser=off  btuserwidth=1  multtype=Use_Mults  optimizegoal=Resources  flowcontrol=NonBlocking  outputwidth=18  roundmode=Truncate  hasctrltlast=off  hasctrltuser=off  ctrltuserwidth=1  outtlastbehv=Null  latencyconfig=Automatic  minimumlatency=37  aclken=off  aresetn=on  trim_axipin_name=on  simulation_type=hybrid_sim  simulation_model=sysgen:cmpy_v6_0  data_path_portlist={ 's_axis_a_tdata_real', 's_axis_a_tdata_imag', 's_axis_b_tdata_real', 's_axis_b_tdata_imag', 's_axis_ctrl_tdata_rounding_bit', 'm_axis_dout_tdata_real', 'm_axis_dout_tdata_imag' }  aportwidth=63  bportwidth=63  ip_name=Complex Multiplier  ip_version=6.0  dsptool_ready=true  ipcore_usecache=true  ipcore_useipmodelcache=true  ipcore_verbose=false  ipcore_latency_parameter='minimumlatency'  wrapper_available=true  port_translation_map={ 'aclken' => 'en', 'aresetn' => 'rst'}  block_type=cmpy_v6_0
  Terminator1 : Terminator
  OutARe : Outport
  OutAIm : Outport  Port=2
  OutBRe : Outport  Port=3
  OutBIm : Outport  Port=4
  LagOut : Outport  Port=5
  Phase : Outport  Port=6
  wires:
  Bipolar NCO/3(phase) -> Phase/1
  Int Offset Mixer/2 -> Convert/1
  Int Offset Mixer/1 -> Phase_Detect/4, Phase_Detect/1
  Conju gate/1 -> Phase_Detect/5
  LagCoef/1 -> LimitedAccum/5(LagCoef)
  LeadCoef/1 -> Mult/2
  Bipolar NCO/2(cos) -> Int Offset Mixer/6
  One/1 -> Int Offset Mixer/1, Int Offset Mixer/4
  Mult/1 -> AddSub/2
  Convert1/1 -> OutBRe/1, Phase_Detect/6
  Phase_Detect/1 -> Terminator1/1
  Convert/1 -> OutBIm/1, Conju gate/1
  Int Offset Mixer/3 -> Convert1/1
  Bipolar NCO/1(sin) -> Int Offset Mixer/5
  Phase_Detect/3 -> Cordic ATan/2(Real)
  Phase_Detect/2 -> Cordic ATan/1(Imag)
  Delay2/1 -> Phase_Detect/2, OutAIm/1
  SecRe/1 -> Int Offset Mixer/3
  Limit/1 -> LimitedAccum/1(Limit)
  SecIm/1 -> Int Offset Mixer/2
  PriRe/1 -> Delay1/1
  PriIm/1 -> Delay2/1
  Delay1/1 -> Phase_Detect/3, OutARe/1
  AddSub/1 -> Negate2/1
  Cordic ATan/1(Phase) -> Negate1/1
  LimitedAccum/1(Out) -> AddSub/1, LagOut/1
  Negate1/1 -> Mult/1, LimitedAccum/2(PhaseErr)
  SwpRate/1 -> LimitedAccum/4(SwpRate)
  [Locked] -> LimitedAccum/3(Locked)
  [Reset] -> Inverter1/1, Bipolar NCO/1(Rst)
  Inverter1/1 -> Phase_Detect/7, Int Offset Mixer/7
  Negate2/1 -> Bipolar NCO/2(Inc)

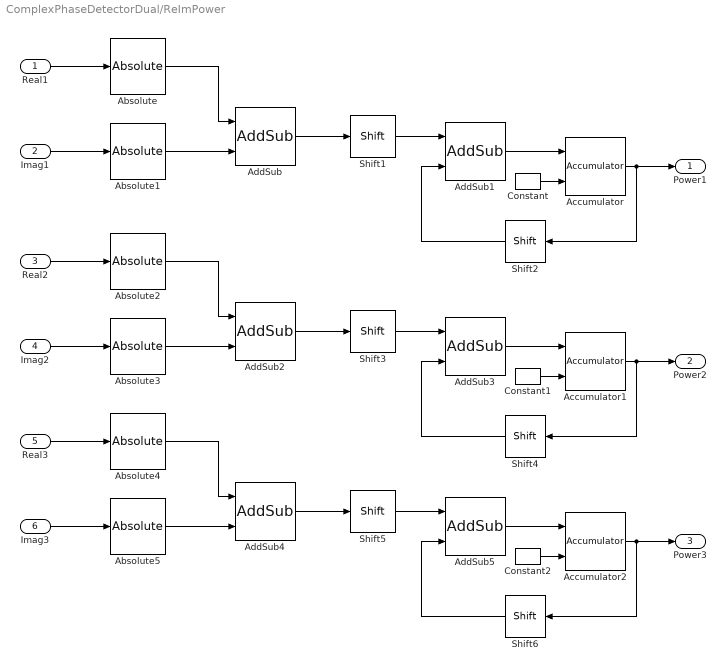
== system ComplexPhaseDetectorDual/ReImPower ==
  Real1 : Inport
  Imag1 : Inport  Port=2
  Real2 : Inport  Port=3
  Imag2 : Inport  Port=4
  Real3 : Inport  Port=5
  Imag3 : Inport  Port=6
  Absolute{,1..5} (6 alike) : xbsIndex_r4/Absolute  precision=Full  arith_type=Unsigned  n_bits=16  bin_pt=14  quantization=Truncate  overflow=Wrap  en=off  latency=0  dbl_ovrd=off  block_type=abs
  Accumulator : xbsIndex_r4/Accumulator  operation=Add  n_bits=21  overflow=Wrap  scale=1  rst=on  hasbypass=off  infoeditControl=reset for floating point data type must be asserted for a minimum of 2 cycles  en=off  latency=1  msb_inp=100  msb=100  lsb=-100  use_behavioral_HDL=on  implementation=Fabric  dbl_ovrd=off  block_type=accum
  Accumulator1 : xbsIndex_r4/Accumulator  operation=Add  n_bits=21  overflow=Wrap  scale=1  rst=on  hasbypass=off  infoeditControl=reset for floating point data type must be asserted for a minimum of 2 cycles  en=off  latency=1  msb_inp=100  msb=100  lsb=-100  use_behavioral_HDL=on  implementation=Fabric  dbl_ovrd=off  block_type=accum
  Accumulator2 : xbsIndex_r4/Accumulator  operation=Add  n_bits=21  overflow=Wrap  scale=1  rst=on  hasbypass=off  infoeditControl=reset for floating point data type must be asserted for a minimum of 2 cycles  en=off  latency=1  msb_inp=100  msb=100  lsb=-100  use_behavioral_HDL=on  implementation=Fabric  dbl_ovrd=off  block_type=accum
  AddSub : xbsIndex_r4/AddSub  mode=Addition  use_carryin=off  use_carryout=off  en=off  latency=1  precision=Full  arith_type=Unsigned  n_bits=16  bin_pt=14  quantization=Truncate  overflow=Wrap  use_behavioral_HDL=off  hw_selection=Fabric  pipelined=off  dbl_ovrd=off  block_type=addsub
  AddSub1 : xbsIndex_r4/AddSub  mode=Subtraction  use_carryin=off  use_carryout=off  en=off  latency=1  precision=Full  arith_type=Unsigned  n_bits=16  bin_pt=14  quantization=Truncate  overflow=Wrap  use_behavioral_HDL=off  hw_selection=Fabric  pipelined=off  dbl_ovrd=off  block_type=addsub
  AddSub2 : xbsIndex_r4/AddSub  mode=Addition  use_carryin=off  use_carryout=off  en=off  latency=1  precision=Full  arith_type=Unsigned  n_bits=16  bin_pt=14  quantization=Truncate  overflow=Wrap  use_behavioral_HDL=off  hw_selection=Fabric  pipelined=off  dbl_ovrd=off  block_type=addsub
  AddSub3 : xbsIndex_r4/AddSub  mode=Subtraction  use_carryin=off  use_carryout=off  en=off  latency=1  precision=Full  arith_type=Unsigned  n_bits=16  bin_pt=14  quantization=Truncate  overflow=Wrap  use_behavioral_HDL=off  hw_selection=Fabric  pipelined=off  dbl_ovrd=off  block_type=addsub
  AddSub4 : xbsIndex_r4/AddSub  mode=Addition  use_carryin=off  use_carryout=off  en=off  latency=1  precision=Full  arith_type=Unsigned  n_bits=16  bin_pt=14  quantization=Truncate  overflow=Wrap  use_behavioral_HDL=off  hw_selection=Fabric  pipelined=off  dbl_ovrd=off  block_type=addsub
  AddSub5 : xbsIndex_r4/AddSub  mode=Subtraction  use_carryin=off  use_carryout=off  en=off  latency=1  precision=Full  arith_type=Unsigned  n_bits=16  bin_pt=14  quantization=Truncate  overflow=Wrap  use_behavioral_HDL=off  hw_selection=Fabric  pipelined=off  dbl_ovrd=off  block_type=addsub
  Constant : xbsIndex_r4/Constant  const=0  gui_display_data_type=Boolean  arith_type=Boolean  n_bits=16  bin_pt=14  preci_type=Single  exp_width=8  frac_width=24  explicit_period=off  period=1  equ=P=C  opselect=C  inp2=PCIN>>17  opr=+  inp1=P  carry=CIN  dbl_ovrd=off  block_type=constant
  Constant1 : xbsIndex_r4/Constant  const=0  gui_display_data_type=Boolean  arith_type=Boolean  n_bits=16  bin_pt=14  preci_type=Single  exp_width=8  frac_width=24  explicit_period=off  period=1  equ=P=C  opselect=C  inp2=PCIN>>17  opr=+  inp1=P  carry=CIN  dbl_ovrd=off  block_type=constant
  Constant2 : xbsIndex_r4/Constant  const=0  gui_display_data_type=Boolean  arith_type=Boolean  n_bits=16  bin_pt=14  preci_type=Single  exp_width=8  frac_width=24  explicit_period=off  period=1  equ=P=C  opselect=C  inp2=PCIN>>17  opr=+  inp1=P  carry=CIN  dbl_ovrd=off  block_type=constant
  Shift{1..6} (6 alike) : xbsIndex_r4/Shift  shift_dir=Right  shift_bits=N  en=off  latency=0  precision=Full  arith_type="Signed  (2's comp)"  n_bits=16  bin_pt=14  quantization=Truncate  overflow=Wrap  dbl_ovrd=off  block_type=shift
  Power1 : Outport
  Power2 : Outport  Port=2
  Power3 : Outport  Port=3
  wires:
  Real1/1 -> Absolute/1
  Imag1/1 -> Absolute1/1
  Accumulator/1 -> Shift2/1, Power1/1
  Absolute/1 -> AddSub/1
  Constant/1 -> Accumulator/2
  Shift2/1 -> AddSub1/2
  Shift1/1 -> AddSub1/1
  Absolute1/1 -> AddSub/2
  AddSub/1 -> Shift1/1
  AddSub1/1 -> Accumulator/1
  Real2/1 -> Absolute2/1
  Imag2/1 -> Absolute3/1
  Accumulator1/1 -> Power2/1, Shift4/1
  Absolute2/1 -> AddSub2/1
  Constant1/1 -> Accumulator1/2
  Shift4/1 -> AddSub3/2
  Shift3/1 -> AddSub3/1
  Absolute3/1 -> AddSub2/2
  AddSub2/1 -> Shift3/1
  AddSub3/1 -> Accumulator1/1
  Real3/1 -> Absolute4/1
  Imag3/1 -> Absolute5/1
  Accumulator2/1 -> Shift6/1, Power3/1
  Absolute4/1 -> AddSub4/1
  Constant2/1 -> Accumulator2/2
  Shift6/1 -> AddSub5/2
  Shift5/1 -> AddSub5/1
  Absolute5/1 -> AddSub4/2
  AddSub4/1 -> Shift5/1
  AddSub5/1 -> Accumulator2/1
